simulink model "tdc_model_02_pid_controller"  (R2018a)
settings: Solver=VariableStepAuto  StartTime=0.0  StopTime=10.0  RelTol=1e-3
undefined symbols (not defined in the file): kp, Td, Ti
settings Model: Creator=aleja  LastModifiedBy=Nicolas

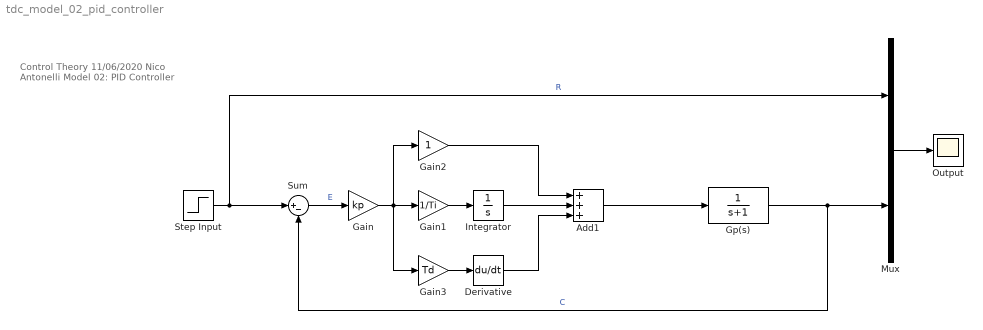
== system tdc_model_02_pid_controller ==
  note: Control Theory
      | 11/06/2020
      | Nico Antonelli
      |
      | Model 02: PID Controller
  Add1 : Sum  Inputs=+++
  Derivative : Derivative  CoefficientInTFapproximation=0.5
  Gain : Gain  Gain=kp
  Gain1 : Gain  Gain=1/Ti
  Gain2 : Gain
  Gain3 : Gain  Gain=Td
  Gp(s) : TransferFcn  Denominator=[1 1]
  Integrator : Integrator  InitialCondition=2
  Mux : Mux  Inputs=2
  Output : Scope
  Step Input : Step  SampleTime=0
  Sum : Sum  Inputs=|+-
  wires:
  Gp(s)/1 -> Mux/2, Sum/2  "C"
  Integrator/1 -> Add1/2
  Gain2/1 -> Add1/1
  Sum/1 -> Gain/1  "E"
  Gain/1 -> Gain3/1, Gain2/1, Gain1/1
  Step Input/1 -> Mux/1, Sum/1  "R"
  Gain1/1 -> Integrator/1
  Gain3/1 -> Derivative/1
  Derivative/1 -> Add1/3
  Mux/1 -> Output/1
  Add1/1 -> Gp(s)/1
